simulink model "Question1"  (R2018b)
settings: Solver=VariableStepAuto  StartTime=0.0  StopTime=100  RelTol=1e-3
libraries: simulink x1
settings Model: Creator=Acer  LastModifiedBy=Acer

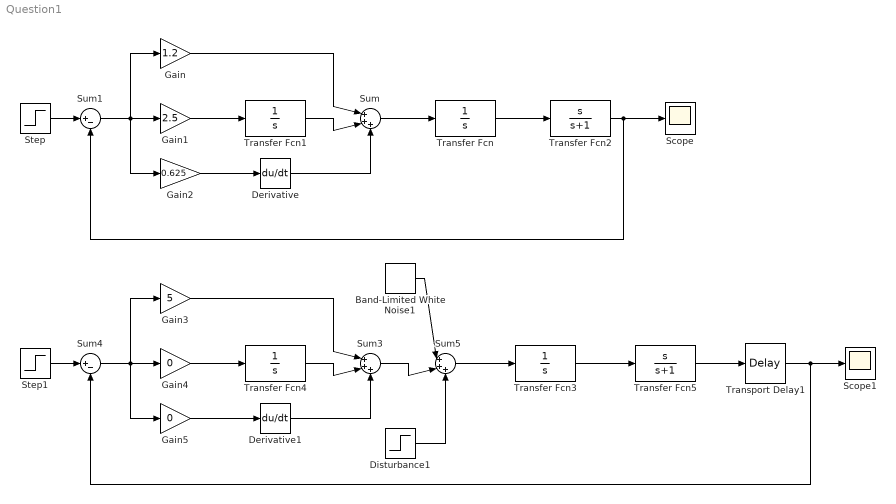
== system Question1 ==
  Band-Limited White Noise1 : simulink/Sources/Band-Limited White Noise  Cov=[0.1]  Ts=0.1  seed=[23341]
  Derivative : Derivative
  Derivative1 : Derivative
  Disturbance1 : Step  SampleTime=0
  Gain : Gain  Gain=1.2
  Gain1 : Gain  Gain=2.5
  Gain2 : Gain  Gain=0.625
  Gain3 : Gain  Gain=5
  Gain4 : Gain  Gain=0
  Gain5 : Gain  Gain=0
  Scope : Scope
  Scope1 : Scope
  Step : Step  SampleTime=0
  Step1 : Step  SampleTime=0
  Sum : Sum  Inputs=|+++
  Sum1 : Sum  Inputs=|+-
  Sum3 : Sum  Inputs=|+++
  Sum4 : Sum  Inputs=|+-
  Sum5 : Sum  Inputs=|+++
  Transfer Fcn{,1,3..4} (4 alike) : TransferFcn  Denominator=[1 0]
  Transfer Fcn2 : TransferFcn  Numerator=[1 0]  Denominator=[1 1]
  Transfer Fcn5 : TransferFcn  Numerator=[1 0]  Denominator=[1 1]
  Transport Delay1 : TransportDelay  DelayTime=0.5
  wires:
  Step/1 -> Sum1/1
  Gain1/1 -> Transfer Fcn1/1
  Gain2/1 -> Derivative/1
  Derivative/1 -> Sum/3
  Gain/1 -> Sum/1
  Transfer Fcn1/1 -> Sum/2
  Sum1/1 -> Gain2/1, Gain/1, Gain1/1
  Transfer Fcn2/1 -> Sum1/2, Scope/1
  Sum/1 -> Transfer Fcn/1
  Transfer Fcn/1 -> Transfer Fcn2/1
  Transfer Fcn3/1 -> Transfer Fcn5/1
  Disturbance1/1 -> Sum5/3
  Derivative1/1 -> Sum3/3
  Transport Delay1/1 -> Sum4/2, Scope1/1
  Sum4/1 -> Gain5/1, Gain3/1, Gain4/1
  Sum5/1 -> Transfer Fcn3/1
  Sum3/1 -> Sum5/2
  Gain3/1 -> Sum3/1
  Transfer Fcn5/1 -> Transport Delay1/1
  Transfer Fcn4/1 -> Sum3/2
  Gain4/1 -> Transfer Fcn4/1
  Step1/1 -> Sum4/1
  Band-Limited White Noise1/1 -> Sum5/1
  Gain5/1 -> Derivative1/1
